simulink model "battery_phfb_inv_single_phase"  (R2024b)
settings: Solver=ode1be  StartTime=0.0  StopTime=simlength  FixedStep=ts_sim  MaxStep=ts_sim
undefined symbols (not defined in the file): Adrso, Aresd, Bresd, Cresd, Crso, dead_time, DThs_init, fPWM_INV, fPWM_ZVS, frequency_grid, I_FS, Iout_dc_nom, ki_i_inv, ki_i_zvs, ki_pll, ki_v_inv, ki_v_zvs, kp_i_inv, kp_i_zvs, kp_pll, kp_v_inv, kp_v_zvs, Ldrso, LFu_dc, magnitude, n1, number_of_cells, Q, q1kalman, q1Kalman, q2kalman, q2Kalman, q3Kalman, RCFu_dc, Rkalman, rKalman, RLFu_dc, Rload, Tambient, tc, ts_inv, ts_zvs, tsample, v1_trafo, v2_trafo, V_FS, Vout_dc_nom, w, weigth
libraries: fl_lib x207, nesl_utility x105, ee_lib x26, cstblocks x7, single_phase_transformer_lib x4, lithium_ion_cell_lib x1, simulink x1
(part 1 of 8)
settings Model: SimulationMode=accelerator  Creator=LTNBDA  LastModifiedBy=dbagn
settings SolverCC: ZeroCrossControl=EnableAll  ZeroCrossAlgorithm=Adaptive  AlgebraicLoopSolver=TrustRegion  SolverResetMethod=Robust  AutoInsertRateTranBlk=on
settings DataIOCC: LimitDataPoints=on  MaxDataPoints=1  SaveFormat=Array  SignalLoggingSaveFormat=ModelDataLogs  SaveOutput=off  SignalLogging=off  DSMLogging=off  SaveTime=off  ReturnWorkspaceOutputs=off
settings OptimizationCC: ExpressionDepthLimit=2147483647  InitFltsAndDblsToZero=on  EfficientMapNaN2IntZero=off  LifeSpan=inf
settings DebuggingCC: SaveWithParameterizedLinksMsg=none  UnderspecifiedInitializationDetection=Classic  MergeDetectMultiDrivingBlocksExec=none  SignalResolutionControl=TryResolveAllWithWarning  SolverPrmCheckMsg=warning  MultiTaskDSMMsg=warning  MultiTaskCondExecSysMsg=none  MultiTaskRateTransMsg=warning  FcnCallInpInsideContextMsg=warning  StateNameClashWarn=warning  SFUnexpectedBacktrackingDiag=warning  SFNoUnconditionalDefaultTransitionDiag=warning  ArithmeticOperatorsInVariantConditions=warning
settings HardwareCC: ProdBitPerLong=64  ProdLargestAtomicFloat=None  ProdIntDivRoundTo=Undefined  ProdEndianess=Unspecified  ProdHWDeviceType=Generic->64-bit Embedded Processor (LP64)  TargetBitPerPointer=64  TargetBitPerSizeT=64  TargetBitPerPtrDiffT=64  TargetLongLongMode=on  TargetIntDivRoundTo=Zero  TargetEndianess=LittleEndian  TargetWordSize=64  TargetHWDeviceType=MATLAB Host  ProdEqTarget=off
settings ModelReferenceCC: EnableRefExpFcnMdlSchedulingChecks=on  PropagateSignalLabelsOutOfModel=off
settings SFSimCC: SimUseLocalCustomCode=off  CustomCodeUndefinedFunction=UseInterfaceOnly
settings RTWCC: RTWUseLocalCustomCode=off  GPUComputeCapability=3.5
settings CodeAppCC: MaxIdLength=128  StateflowObjectComments=on
settings GRTTargetCC: TargetLangStandard=C89/C90 (ANSI)  CombineOutputUpdateFcns=off  GRTInterface=on
settings ConfigComp: CovMetricSettings=dw  CovSaveCumulativeToWorkspaceVar=on  CovSaveSingleToWorkspaceVar=on  CovExternalEMLEnable=off
settings SimscapeCC: SimscapeNormalizeSystem=off

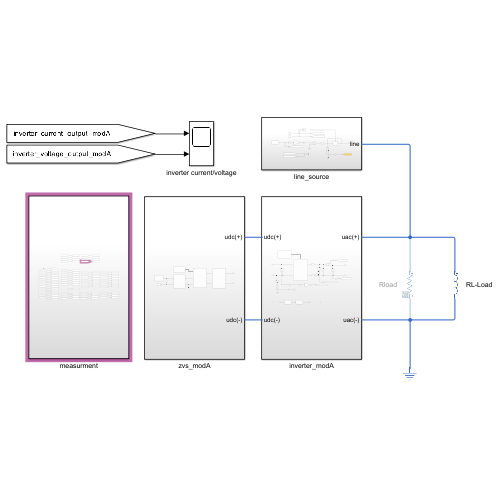
[thumbnail: Simulink's stored preview of the top-level diagram]
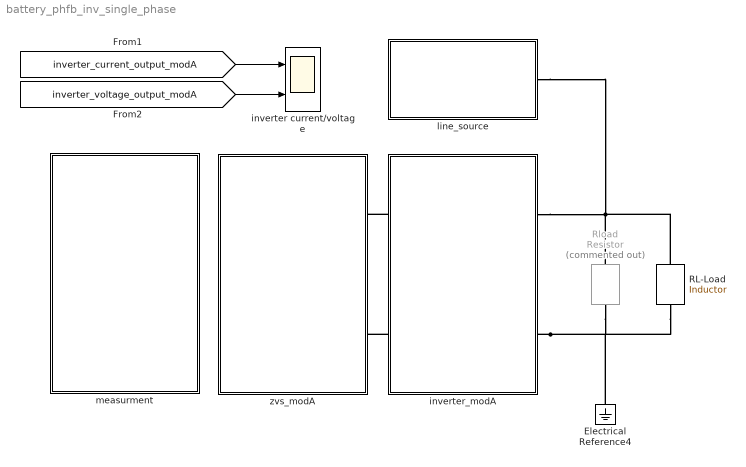
== system battery_phfb_inv_single_phase ==
  Electrical Reference4 : fl_lib/Electrical/Electrical Elements/Electrical Reference
  RL-Load : fl_lib/Electrical/Electrical Elements/Inductor  l=Lload H  r=Rload Ohm  g=1e-9 1/Ohm  i_specify=off  i_priority=None  i=0 A  i_nominal_specify=off  i_nominal_value=1  i_nominal_unit=A  v_specify=off  v_priority=None  v=0 V  v_nominal_specify=off  v_nominal_value=1  v_nominal_unit=V  i_L_specify=off  i_L_priority=High  i_L=0 A  i_L_nominal_specify=off  i_L_nominal_value=1  i_L_nominal_unit=A
  Rload : fl_lib/Electrical/Electrical Elements/Resistor  Commented=on  R=Rload Ohm  i_specify=off  i_priority=None  i=0 A  i_nominal_specify=off  i_nominal_value=1  i_nominal_unit=A  v_specify=off  v_priority=None  v=0 V  v_nominal_specify=off  v_nominal_value=1  v_nominal_unit=V
  inverter current/voltage : Scope  NumInputPorts=2
  inverter_modA : Subsystem
  line_source : Subsystem
  measurment : Subsystem
  zvs_modA : Subsystem
  wires:
  [inverter_current_output_modA] -> inverter current/voltage/1
  [inverter_voltage_output_modA] -> inverter current/voltage/2
  connections:
  inverter_modA/LConn2 -- zvs_modA/RConn2
  inverter_modA/LConn1 -- zvs_modA/RConn1
  inverter_modA/RConn1 -- RL-Load/LConn1 -- Rload/LConn1 -- line_source/LConn1
  inverter_modA/RConn2 -- RL-Load/RConn1 -- Rload/RConn1 -- Electrical Reference4/LConn1

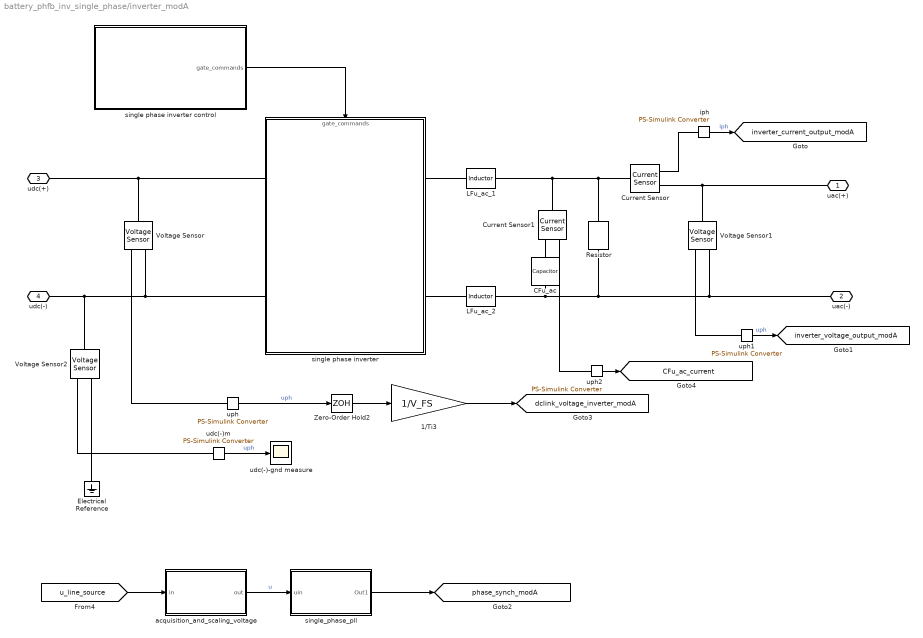
== system battery_phfb_inv_single_phase/inverter_modA ==
  1/Ti3 : Gain  Gain=1/V_FS  SaturateOnIntegerOverflow=on  OutDataTypeStr=Inherit: Same as input  ParamDataTypeStr=Inherit: Same as input
  CFu_ac : fl_lib/Electrical/Electrical Elements/Capacitor  c=CFu_ac F  r=RCFu_ac Ohm  g=0 1/Ohm  i_specify=off  i_priority=None  i=0 A  i_nominal_specify=off  i_nominal_value=1  i_nominal_unit=A  v_specify=off  v_priority=None  v=0 V  v_nominal_specify=off  v_nominal_value=1  v_nominal_unit=V  vc_specify=off  vc_priority=High  vc=0 V  vc_nominal_specify=off  vc_nominal_value=1  vc_nominal_unit=V
  Current Sensor : fl_lib/Electrical/Electrical Sensors/Current Sensor
  Current Sensor1 : fl_lib/Electrical/Electrical Sensors/Current Sensor
  Electrical Reference : fl_lib/Electrical/Electrical Elements/Electrical Reference
  LFu_ac_1 : fl_lib/Electrical/Electrical Elements/Inductor  l=LFu_ac H  r=RLFu_ac Ohm  g=0 1/Ohm  i_specify=off  i_priority=None  i=0 A  i_nominal_specify=off  i_nominal_value=1  i_nominal_unit=A  v_specify=off  v_priority=None  v=0 V  v_nominal_specify=off  v_nominal_value=1  v_nominal_unit=V  i_L_specify=off  i_L_priority=High  i_L=0 A  i_L_nominal_specify=off  i_L_nominal_value=1  i_L_nominal_unit=A
  LFu_ac_2 : fl_lib/Electrical/Electrical Elements/Inductor  l=LFu_ac H  r=RLFu_ac Ohm  g=0 1/Ohm  i_specify=off  i_priority=None  i=0 A  i_nominal_specify=off  i_nominal_value=1  i_nominal_unit=A  v_specify=off  v_priority=None  v=0 V  v_nominal_specify=off  v_nominal_value=1  v_nominal_unit=V  i_L_specify=off  i_L_priority=High  i_L=0 A  i_L_nominal_specify=off  i_L_nominal_value=1  i_L_nominal_unit=A
  Resistor : fl_lib/Electrical/Electrical Elements/Resistor  R=10e3 Ohm  i_specify=off  i_priority=None  i=0 A  i_nominal_specify=off  i_nominal_value=1  i_nominal_unit=A  v_specify=off  v_priority=None  v=0 V  v_nominal_specify=off  v_nominal_value=1  v_nominal_unit=V
  Voltage Sensor : fl_lib/Electrical/Electrical Sensors/Voltage Sensor
  Voltage Sensor1 : fl_lib/Electrical/Electrical Sensors/Voltage Sensor
  Voltage Sensor2 : fl_lib/Electrical/Electrical Sensors/Voltage Sensor
  Zero-Order Hold2 : ZeroOrderHold  SampleTime=ts_zvs
  acquisition_and_scaling_voltage : Subsystem
  iph : nesl_utility/PS-Simulink Converter  PhysicalDomain=network_engine_domain  SubClassName=ps_output  LeftPortType=input  RightPortType=output  PseudoPeriodic=off  Frequencies=[]  VectorFormat=1-D array  Unit=A  AffineConversion=off
  single phase inverter : Subsystem
      settings: PortSchema="{\"entries\":[{\"content\":{\"sides\":[{\"content\":{\"connectorIds\":[\"LConn1\",\"LConn2\"]},\"type\":\"ConnectorPlacement.EquallySpacedRectSide\",\"uuid\":\"4fcf4fea-d38f-431b-8a91-be3ce9782faf\"},{\"content\":{\"connectorIds\":[\"RConn1\",\"RConn2\"],\"side\":\"RIGHT\"},\"type\":\"ConnectorPlacement.EquallySpacedRectSide\",\"uuid\":\"0aa56277-92e9-4e3b-84c7-43398254a4d8\"},{\"content\":{\"connectorIds\":[\"In1\"],\"side\":\"TOP\"},\"type\":\"ConnectorPlacement.EquallySpacedRectSide\",\"uuid\":\"5cd150dc-bcaf-4cd7-b2a8-3db203726730\"}]},\"type\":\"ConnectorPlacement.EquallySpacedConnector\",\"uuid\":\"bf8194c4-c327-4d40-bea4-f1e7617f80b4\"}],\"packageUris\":[\"http://schema.mathworks.com/mf0/Connector/R2020b\"],\"version\":\"1.0\"}"
  single phase inverter control : Subsystem
  single_phase_pll : Subsystem
  udc(-)-gnd measure : Scope
  udc(-)m : nesl_utility/PS-Simulink Converter  PhysicalDomain=network_engine_domain  SubClassName=ps_output  LeftPortType=input  RightPortType=output  PseudoPeriodic=off  Frequencies=[]  VectorFormat=1-D array  Unit=V  AffineConversion=off
  uph : nesl_utility/PS-Simulink Converter  PhysicalDomain=network_engine_domain  SubClassName=ps_output  LeftPortType=input  RightPortType=output  PseudoPeriodic=off  Frequencies=[]  VectorFormat=1-D array  Unit=V  AffineConversion=off
  uph1 : nesl_utility/PS-Simulink Converter  PhysicalDomain=network_engine_domain  SubClassName=ps_output  LeftPortType=input  RightPortType=output  PseudoPeriodic=off  Frequencies=[]  VectorFormat=1-D array  Unit=V  AffineConversion=off
  uph2 : nesl_utility/PS-Simulink Converter  PhysicalDomain=network_engine_domain  SubClassName=ps_output  LeftPortType=input  RightPortType=output  PseudoPeriodic=off  Frequencies=[]  VectorFormat=1-D array  Unit=A  AffineConversion=off
  uac(+) : PMIOPort  Side=Right
  uac(-) : PMIOPort  Port=2  Side=Right
  udc(+) : PMIOPort  Port=3  Side=Left
  udc(-) : PMIOPort  Port=4  Side=Left
  tag scope: CFu_ac_current=global, dclink_voltage_inverter_modA=global, inverter_current_output_modA=global, inverter_voltage_output_modA=global, phase_synch_modA=global
  wires:
  single phase inverter control/1(gate_commands) -> single phase inverter/1(gate_commands)
  iph/1 -> [inverter_current_output_modA]  "iph"
  uph1/1 -> [inverter_voltage_output_modA]  "uph"
  uph2/1 -> [CFu_ac_current]
  acquisition_and_scaling_voltage/1(out) -> single_phase_pll/1(uin)  "u"
  single_phase_pll/1(Out1) -> [phase_synch_modA]
  [u_line_source] -> acquisition_and_scaling_voltage/1(in)
  uph/1 -> Zero-Order Hold2/1  "uph"
  Zero-Order Hold2/1 -> 1/Ti3/1
  udc(-)m/1 -> udc(-)-gnd measure/1  "uph"
  1/Ti3/1 -> [dclink_voltage_inverter_modA]
  connections:
  single phase inverter/RConn2 -- Voltage Sensor2/LConn1 -- udc(-)/RConn1 -- Voltage Sensor/RConn2
  single phase inverter/RConn1 -- Voltage Sensor/LConn1 -- udc(+)/RConn1
  LFu_ac_1/LConn1 -- single phase inverter/LConn1
  single phase inverter/LConn2 -- LFu_ac_2/RConn1
  Voltage Sensor1/RConn1 -- uph1/LConn1
  Resistor/LConn1 -- Current Sensor/LConn1 -- Current Sensor1/LConn1 -- LFu_ac_1/RConn1
  iph/LConn1 -- Current Sensor/RConn1
  Current Sensor/RConn2 -- uac(+)/RConn1 -- Voltage Sensor1/LConn1
  LFu_ac_2/LConn1 -- CFu_ac/RConn1 -- uac(-)/RConn1 -- Voltage Sensor1/RConn2 -- Resistor/RConn1
  Current Sensor1/RConn2 -- CFu_ac/LConn1
  Current Sensor1/RConn1 -- uph2/LConn1
  Electrical Reference/LConn1 -- Voltage Sensor2/RConn2
  Voltage Sensor2/RConn1 -- udc(-)m/LConn1
  Voltage Sensor/RConn1 -- uph/LConn1

== system battery_phfb_inv_single_phase/line_source ==
  Controlled Voltage Source : fl_lib/Electrical/Electrical Sources/Controlled Voltage Source
  Cos : Trigonometry  Operator=cos
  Electrical Reference : fl_lib/Electrical/Electrical Elements/Electrical Reference
  Electrical Reference1 : fl_lib/Electrical/Electrical Elements/Electrical Reference
  Gain : Gain  Gain=230*sqrt(2)
  Ld_grid : fl_lib/Electrical/Electrical Elements/Inductor  l=250e-6 H  r=3e-3 Ohm  g=0 1/Ohm  i_specify=off  i_priority=None  i=0 A  i_nominal_specify=off  i_nominal_value=1  i_nominal_unit=A  v_specify=off  v_priority=None  v=0 V  v_nominal_specify=off  v_nominal_value=1  v_nominal_unit=V  i_L_specify=off  i_L_priority=High  i_L=0 A  i_L_nominal_specify=off  i_L_nominal_value=1  i_L_nominal_unit=A
  Simulink-PS Converter : nesl_utility/Simulink-PS Converter  PhysicalDomain=network_engine_domain  SubClassName=ps_input  LeftPortType=input  RightPortType=output  PseudoPeriodic=off  Frequencies=[]  NoiseDistribution=none  NoiseParameters=[]  Unit=1  AffineConversion=off  FilteringAndDerivatives=provide  SimscapeFilterOrder=1  InputFilterTimeConstant=0.001  UdotUserProvided=0
  Step : Step  Time=2e3  After=15  SampleTime=0
  Step1 : Step  Time=1.2  Before=15  After=0  SampleTime=0
  Voltage Sensor2 : fl_lib/Electrical/Electrical Sensors/Voltage Sensor
  cmd_bypass_line/ups : Scope  NumInputPorts=2
  ideas_switch_based_switch1 : Subsystem
      settings: PortSchema="{\"entries\":[{\"content\":{\"sides\":[{\"content\":{\"connectorIds\":[\"LConn1\"]},\"type\":\"ConnectorPlacement.EquallySpacedRectSide\",\"uuid\":\"0c1d3d49-2b2f-458b-aa4f-29a8fc7e06a8\"},{\"content\":{\"connectorIds\":[\"RConn1\"],\"side\":\"RIGHT\"},\"type\":\"ConnectorPlacement.EquallySpacedRectSide\",\"uuid\":\"ca3eb42d-18fc-4989-b764-44975cb49bad\"},{\"content\":{\"connectorIds\":[\"In1\"],\"side\":\"TOP\"},\"type\":\"ConnectorPlacement.EquallySpacedRectSide\",\"uuid\":\"521c1188-cf36-48df-a46f-4a5e2a9fee19\"}]},\"type\":\"ConnectorPlacement.EquallySpacedConnector\",\"uuid\":\"019ba21c-6ae7-40bf-b23d-41e1cbba37d5\"}],\"packageUris\":[\"http://schema.mathworks.com/mf0/Connector/R2020b\"],\"version\":\"1.0\"}"
  phase_gen : Subsystem
  phase_grid/pll : Scope  NumInputPorts=2
  u_line_source : nesl_utility/PS-Simulink Converter  PhysicalDomain=network_engine_domain  SubClassName=ps_output  LeftPortType=input  RightPortType=output  PseudoPeriodic=off  Frequencies=[]  VectorFormat=1-D array  Unit=V  AffineConversion=off
  line : PMIOPort  Side=Left
  tag scope: cmd_bypass_line=global, cmd_bypass_ups=global, phase_grid=global, u_line_source=global
  wires:
  phase_gen/1(phase_gen) -> Cos/1, [phase_grid]
  Step1/1 -> cmd_bypass_line/ups/2, [cmd_bypass_ups]  "cmd_bypass_ups"
  Step/1 -> cmd_bypass_line/ups/1, [cmd_bypass_line]  "cmd_bypass_line"
  Cos/1 -> Gain/1
  Gain/1 -> Simulink-PS Converter/1
  [phase_synch_modA] -> phase_grid/pll/1  "phase_synch_modA"
  [phase_grid] -> phase_grid/pll/2  "phase_grid"
  [cmd_bypass_line] -> ideas_switch_based_switch1/1(gate_firing)
  u_line_source/1 -> [u_line_source]  "u_line_source"
  connections:
  Simulink-PS Converter/RConn1 -- Controlled Voltage Source/RConn1
  Electrical Reference/LConn1 -- Controlled Voltage Source/RConn2
  Controlled Voltage Source/LConn1 -- Ld_grid/LConn1
  Ld_grid/RConn1 -- ideas_switch_based_switch1/LConn1
  ideas_switch_based_switch1/RConn1 -- line/RConn1 -- Voltage Sensor2/LConn1
  Voltage Sensor2/RConn1 -- u_line_source/LConn1
  Electrical Reference1/LConn1 -- Voltage Sensor2/RConn2

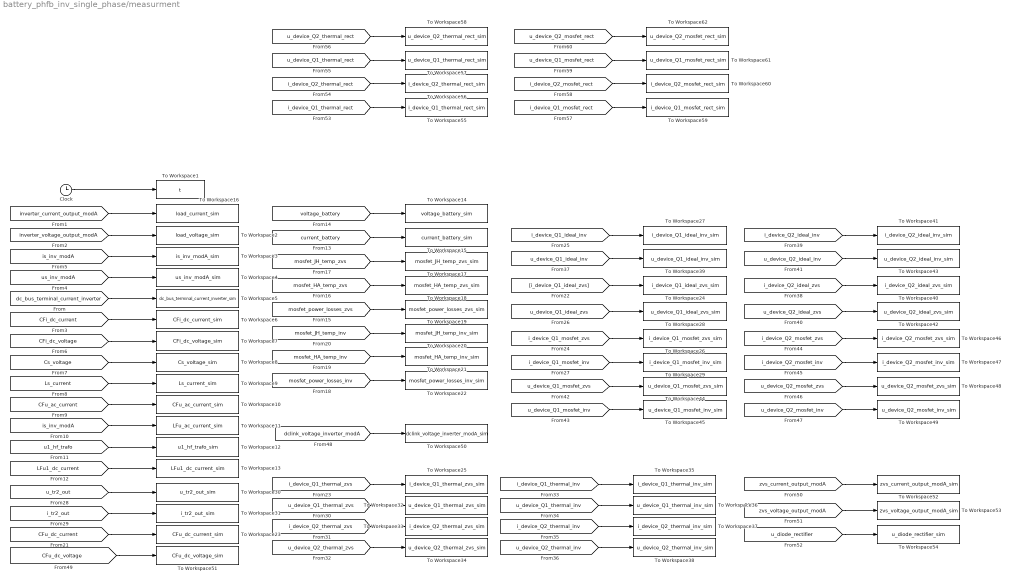
== system battery_phfb_inv_single_phase/measurment ==
  Clock : Clock
  To Workspace1 : ToWorkspace  VariableName=t  SampleTime=tc
      settings: MaxDataPoints=Nc
  To Workspace10 : ToWorkspace  VariableName=CFu_ac_current_sim  SampleTime=tc
      settings: MaxDataPoints=Nc
  To Workspace11 : ToWorkspace  VariableName=LFu_ac_current_sim  SampleTime=tc
      settings: MaxDataPoints=Nc
  To Workspace12 : ToWorkspace  VariableName=u1_hf_trafo_sim  SampleTime=tc
      settings: MaxDataPoints=Nc
  To Workspace13 : ToWorkspace  VariableName=LFu1_dc_current_sim  SampleTime=tc
      settings: MaxDataPoints=Nc
  To Workspace14 : ToWorkspace  VariableName=voltage_battery_sim  SampleTime=tc
      settings: MaxDataPoints=Nc
  To Workspace15 : ToWorkspace  VariableName=current_battery_sim  SampleTime=tc
      settings: MaxDataPoints=Nc
  To Workspace16 : ToWorkspace  VariableName=load_current_sim  SampleTime=tc
      settings: MaxDataPoints=Nc
  To Workspace17 : ToWorkspace  VariableName=mosfet_JH_temp_zvs_sim  SampleTime=tc
      settings: MaxDataPoints=Nc
  To Workspace18 : ToWorkspace  VariableName=mosfet_HA_temp_zvs_sim  SampleTime=tc
      settings: MaxDataPoints=Nc
  To Workspace19 : ToWorkspace  VariableName=mosfet_power_losses_zvs_sim  SampleTime=tc
      settings: MaxDataPoints=Nc
  To Workspace2 : ToWorkspace  VariableName=load_voltage_sim  SampleTime=tc
      settings: MaxDataPoints=Nc
  To Workspace20 : ToWorkspace  VariableName=mosfet_JH_temp_inv_sim  SampleTime=tc
      settings: MaxDataPoints=Nc
  To Workspace21 : ToWorkspace  VariableName=mosfet_HA_temp_inv_sim  SampleTime=tc
      settings: MaxDataPoints=Nc
  To Workspace22 : ToWorkspace  VariableName=mosfet_power_losses_inv_sim  SampleTime=tc
      settings: MaxDataPoints=Nc
  To Workspace23 : ToWorkspace  VariableName=CFu_dc_current_sim  SampleTime=tc
      settings: MaxDataPoints=Nc
  To Workspace24 : ToWorkspace  VariableName=i_device_Q1_ideal_zvs_sim  SampleTime=tc
      settings: MaxDataPoints=Nc
  To Workspace25 : ToWorkspace  VariableName=i_device_Q1_thermal_zvs_sim  SampleTime=tc
      settings: MaxDataPoints=Nc
  To Workspace26 : ToWorkspace  VariableName=i_device_Q1_mosfet_zvs_sim  SampleTime=tc
      settings: MaxDataPoints=Nc
  To Workspace27 : ToWorkspace  VariableName=i_device_Q1_ideal_inv_sim  SampleTime=tc
      settings: MaxDataPoints=Nc
  To Workspace28 : ToWorkspace  VariableName=u_device_Q1_ideal_zvs_sim  SampleTime=tc
      settings: MaxDataPoints=Nc
  To Workspace29 : ToWorkspace  VariableName=i_device_Q1_mosfet_inv_sim  SampleTime=tc
      settings: MaxDataPoints=Nc
  To Workspace3 : ToWorkspace  VariableName=is_inv_modA_sim  SampleTime=tc
      settings: MaxDataPoints=Nc
  To Workspace30 : ToWorkspace  VariableName=u_tr2_out_sim  SampleTime=tc
      settings: MaxDataPoints=Nc
  To Workspace31 : ToWorkspace  VariableName=i_tr2_out_sim  SampleTime=tc
      settings: MaxDataPoints=Nc
  To Workspace32 : ToWorkspace  VariableName=u_device_Q1_thermal_zvs_sim  SampleTime=tc
      settings: MaxDataPoints=Nc
  To Workspace33 : ToWorkspace  VariableName=i_device_Q2_thermal_zvs_sim  SampleTime=tc
      settings: MaxDataPoints=Nc
  To Workspace34 : ToWorkspace  VariableName=u_device_Q2_thermal_zvs_sim  SampleTime=tc
      settings: MaxDataPoints=Nc
  To Workspace35 : ToWorkspace  VariableName=i_device_Q1_thermal_inv_sim  SampleTime=tc
      settings: MaxDataPoints=Nc
  To Workspace36 : ToWorkspace  VariableName=u_device_Q1_thermal_inv_sim  SampleTime=tc
      settings: MaxDataPoints=Nc
  To Workspace37 : ToWorkspace  VariableName=i_device_Q2_thermal_inv_sim  SampleTime=tc
      settings: MaxDataPoints=Nc
  To Workspace38 : ToWorkspace  VariableName=u_device_Q2_thermal_inv_sim  SampleTime=tc
      settings: MaxDataPoints=Nc
  To Workspace39 : ToWorkspace  VariableName=u_device_Q1_ideal_inv_sim  SampleTime=tc
      settings: MaxDataPoints=Nc
  To Workspace4 : ToWorkspace  VariableName=us_inv_modA_sim  SampleTime=tc
      settings: MaxDataPoints=Nc
  To Workspace40 : ToWorkspace  VariableName=i_device_Q2_ideal_zvs_sim  SampleTime=tc
      settings: MaxDataPoints=Nc
  To Workspace41 : ToWorkspace  VariableName=i_device_Q2_ideal_inv_sim  SampleTime=tc
      settings: MaxDataPoints=Nc
  To Workspace42 : ToWorkspace  VariableName=u_device_Q2_ideal_zvs_sim  SampleTime=tc
      settings: MaxDataPoints=Nc
  To Workspace43 : ToWorkspace  VariableName=u_device_Q2_ideal_inv_sim  SampleTime=tc
      settings: MaxDataPoints=Nc
  To Workspace44 : ToWorkspace  VariableName=u_device_Q1_mosfet_zvs_sim  SampleTime=tc
      settings: MaxDataPoints=Nc
  To Workspace45 : ToWorkspace  VariableName=u_device_Q1_mosfet_inv_sim  SampleTime=tc
      settings: MaxDataPoints=Nc
  To Workspace46 : ToWorkspace  VariableName=i_device_Q2_mosfet_zvs_sim  SampleTime=tc
      settings: MaxDataPoints=Nc
  To Workspace47 : ToWorkspace  VariableName=i_device_Q2_mosfet_inv_sim  SampleTime=tc
      settings: MaxDataPoints=Nc
  To Workspace48 : ToWorkspace  VariableName=u_device_Q2_mosfet_zvs_sim  SampleTime=tc
      settings: MaxDataPoints=Nc
  To Workspace49 : ToWorkspace  VariableName=u_device_Q2_mosfet_inv_sim  SampleTime=tc
      settings: MaxDataPoints=Nc
  To Workspace5 : ToWorkspace  VariableName=dc_bus_terminal_current_inverter_sim  SampleTime=tc
      settings: MaxDataPoints=Nc
  To Workspace50 : ToWorkspace  VariableName=dclink_voltage_inverter_modA_sim  SampleTime=tc
      settings: MaxDataPoints=Nc
  To Workspace51 : ToWorkspace  VariableName=CFu_dc_voltage_sim  SampleTime=tc
      settings: MaxDataPoints=Nc
  To Workspace52 : ToWorkspace  VariableName=zvs_current_output_modA_sim  SampleTime=tc
      settings: MaxDataPoints=Nc
  To Workspace53 : ToWorkspace  VariableName=zvs_voltage_output_modA_sim  SampleTime=tc
      settings: MaxDataPoints=Nc
  To Workspace54 : ToWorkspace  VariableName=u_diode_rectifier_sim  SampleTime=tc
      settings: MaxDataPoints=Nc
  To Workspace55 : ToWorkspace  VariableName=i_device_Q1_thermal_rect_sim  SampleTime=tc
      settings: MaxDataPoints=Nc
  To Workspace56 : ToWorkspace  VariableName=i_device_Q2_thermal_rect_sim  SampleTime=tc
      settings: MaxDataPoints=Nc
  To Workspace57 : ToWorkspace  VariableName=u_device_Q1_thermal_rect_sim  SampleTime=tc
      settings: MaxDataPoints=Nc
  To Workspace58 : ToWorkspace  VariableName=u_device_Q2_thermal_rect_sim  SampleTime=tc
      settings: MaxDataPoints=Nc
  To Workspace59 : ToWorkspace  VariableName=i_device_Q1_mosfet_rect_sim  SampleTime=tc
      settings: MaxDataPoints=Nc
  To Workspace6 : ToWorkspace  VariableName=CFi_dc_current_sim  SampleTime=tc
      settings: MaxDataPoints=Nc
  To Workspace60 : ToWorkspace  VariableName=i_device_Q2_mosfet_rect_sim  SampleTime=tc
      settings: MaxDataPoints=Nc
  To Workspace61 : ToWorkspace  VariableName=u_device_Q1_mosfet_rect_sim  SampleTime=tc
      settings: MaxDataPoints=Nc
  To Workspace62 : ToWorkspace  VariableName=u_device_Q2_mosfet_rect_sim  SampleTime=tc
      settings: MaxDataPoints=Nc
  To Workspace7 : ToWorkspace  VariableName=CFi_dc_voltage_sim  SampleTime=tc
      settings: MaxDataPoints=Nc
  To Workspace8 : ToWorkspace  VariableName=Cs_voltage_sim  SampleTime=tc
      settings: MaxDataPoints=Nc
  To Workspace9 : ToWorkspace  VariableName=Ls_current_sim  SampleTime=tc
      settings: MaxDataPoints=Nc
  wires:
  Clock/1 -> To Workspace1/1
  [inverter_current_output_modA] -> To Workspace16/1
  [inverter_voltage_output_modA] -> To Workspace2/1
  [is_inv_modA] -> To Workspace3/1
  [us_inv_modA] -> To Workspace4/1
  [dc_bus_terminal_current_inverter] -> To Workspace5/1
  [CFi_dc_current] -> To Workspace6/1
  [CFi_dc_voltage] -> To Workspace7/1
  [Cs_voltage] -> To Workspace8/1
  [Ls_current] -> To Workspace9/1
  [CFu_ac_current] -> To Workspace10/1
  [is_inv_modA] -> To Workspace11/1
  [u1_hf_trafo] -> To Workspace12/1
  [LFu1_dc_current] -> To Workspace13/1
  [voltage_battery] -> To Workspace14/1
  [current_battery] -> To Workspace15/1
  [mosfet_JH_temp_zvs] -> To Workspace17/1
  [mosfet_HA_temp_zvs] -> To Workspace18/1
  [mosfet_power_losses_zvs] -> To Workspace19/1
  [mosfet_power_losses_inv] -> To Workspace22/1
  [mosfet_HA_temp_inv] -> To Workspace21/1
  [mosfet_JH_temp_inv] -> To Workspace20/1
  [CFu_dc_current] -> To Workspace23/1
  [i_device_Q1_ideal_zvs] -> To Workspace24/1
  [i_device_Q1_thermal_zvs] -> To Workspace25/1
  [i_device_Q1_mosfet_zvs] -> To Workspace26/1
  [i_device_Q1_mosfet_inv] -> To Workspace29/1
  [i_device_Q1_ideal_inv] -> To Workspace27/1
  [u_tr2_out] -> To Workspace30/1
  [i_tr2_out] -> To Workspace31/1
  [u_device_Q1_thermal_zvs] -> To Workspace32/1
  [u_device_Q2_thermal_zvs] -> To Workspace34/1
  [i_device_Q2_thermal_zvs] -> To Workspace33/1
  [i_device_Q2_thermal_inv] -> To Workspace37/1
  [u_device_Q2_thermal_inv] -> To Workspace38/1
  [u_device_Q1_thermal_inv] -> To Workspace36/1
  [i_device_Q1_thermal_inv] -> To Workspace35/1
  [u_device_Q1_ideal_zvs] -> To Workspace28/1
  [u_device_Q1_ideal_inv] -> To Workspace39/1
  [u_device_Q2_ideal_inv] -> To Workspace43/1
  [u_device_Q2_ideal_zvs] -> To Workspace42/1
  [i_device_Q2_ideal_inv] -> To Workspace41/1
  [i_device_Q2_ideal_zvs] -> To Workspace40/1
  [u_device_Q1_mosfet_inv] -> To Workspace45/1
  [u_device_Q1_mosfet_zvs] -> To Workspace44/1
  [u_device_Q2_mosfet_zvs] -> To Workspace48/1
  [u_device_Q2_mosfet_inv] -> To Workspace49/1
  [i_device_Q2_mosfet_inv] -> To Workspace47/1
  [i_device_Q2_mosfet_zvs] -> To Workspace46/1
  [dclink_voltage_inverter_modA] -> To Workspace50/1
  [CFu_dc_voltage] -> To Workspace51/1
  [zvs_voltage_output_modA] -> To Workspace53/1
  [zvs_current_output_modA] -> To Workspace52/1
  [u_diode_rectifier] -> To Workspace54/1
  [i_device_Q1_thermal_rect] -> To Workspace55/1
  [i_device_Q2_thermal_rect] -> To Workspace56/1
  [u_device_Q2_thermal_rect] -> To Workspace58/1
  [u_device_Q1_thermal_rect] -> To Workspace57/1
  [u_device_Q1_mosfet_rect] -> To Workspace61/1
  [u_device_Q2_mosfet_rect] -> To Workspace62/1
  [i_device_Q2_mosfet_rect] -> To Workspace60/1
  [i_device_Q1_mosfet_rect] -> To Workspace59/1

== system battery_phfb_inv_single_phase/zvs_modA ==
  Electrical Reference : fl_lib/Electrical/Electrical Elements/Electrical Reference
  Solver Configuration : nesl_utility/Solver Configuration  PhysicalDomain=network_engine_domain  SubClassName=solver  LeftPortType=input  RightPortType=generic  Tones=[]  Harmonics=[]  SimulateNoise=off  Profile=off  UseLocalSampling=off  EnableSwitchedLinearOptims=on  FrequencyDomain=off  UseCCode=off  RelTol=0.001  AbsTol=0.001  MinStep=1e-09  ToWorkspace=off  RevertToSquareIcSolve=off  NumHomotopyIterations=100  PhasorMode=off  PhasorModeNumHarmonics=1  ConsistencySolver=NEWTON_FTOL  IndexReductionMethod=DerivativeReplacement  DoDC=on  ResidualTolerance=1e-09  ConsistencyTolSource=GLOBAL  ConsistencyAbsTol=0.001  ConsistencyRelTol=0.001  ConsistencyTolFactor=0.001  UseLocalSolver=on  LocalSolverChoice=NE_BACKWARD_EULER_ADVANCER  ResolveIndetEquations=on  FunctionEvalNumThread=1  LocalSolverSampleTime=ts_sim  DoFixedCost=on  MaxNonlinIter=3  MaxModeIter=2  ComputeImpulses=off  ImpulseIterations=2  LinearAlgebra=auto  LinearAlgebraNumThread=0  EquationFormulation=NE_TIME_EF  DelaysMemoryBudget=1024  AutomaticFiltering=on  FilteringTimeConstant=0.001  PartitionStorageMethod=AS_NEEDED  PartitionMemoryBudget=1024  PartitionMethod=ROBUST  MultibodyUseLocalSolver=off  MultibodyLocalSolverChoice=ODE1  MultibodyLocalSolverSampleTime=0.001
  Voltage Source : ee_lib/Sources/Voltage Source  Commented=on  dc_voltage=90 V  ac_voltage=0 V  ac_shift=0 rad  ac_frequency=60 Hz  noise_mode=ee.enum.sources.noise.Disabled  PSD=0 V^2/Hz  sample_time=1e-3 s  repeatability=ee.enum.sources.repeatability.NotRepeatable  user_seed=0  auto_seed=3499211588  i_specify=off  i_priority=None  i=0 A  i_nominal_specify=off  i_nominal_value=1  i_nominal_unit=A  v_specify=off  v_priority=None  v=0 V  v_nominal_specify=off  v_nominal_value=1  v_nominal_unit=V
  battery_system : Subsystem
  dc/dc with galvanic isolation : Subsystem
  single_phase_ui_measure1 : Subsystem
  ui_measure : Subsystem
  zvs_ctrl : Subsystem
  udc(+) : PMIOPort  Side=Right
  udc(-) : PMIOPort  Port=2  Side=Right
  wires:
  zvs_ctrl/1(gate_commands) -> dc/dc with galvanic isolation/1(gate_commands)
  connections:
  dc/dc with galvanic isolation/RConn1 -- ui_measure/LConn1
  dc/dc with galvanic isolation/RConn2 -- ui_measure/LConn2
  udc(+)/RConn1 -- ui_measure/RConn1
  udc(-)/RConn1 -- ui_measure/RConn2
  dc/dc with galvanic isolation/LConn2 -- single_phase_ui_measure1/RConn2 -- Electrical Reference/LConn1
  battery_system/RConn1 -- Voltage Source/LConn1 -- single_phase_ui_measure1/LConn1
  single_phase_ui_measure1/RConn1 -- dc/dc with galvanic isolation/LConn1
  single_phase_ui_measure1/LConn2 -- Voltage Source/RConn1 -- Solver Configuration/RConn1

== system battery_phfb_inv_single_phase/inverter_modA/acquisition_and_scaling_voltage ==
  in : Inport
  1/Ti1 : Gain  Gain=1/V_FS  SaturateOnIntegerOverflow=on  OutDataTypeStr=Inherit: Same as input  ParamDataTypeStr=Inherit: Same as input
  Unit Delay4 : UnitDelay  SampleTime=ts_inv  HasFrameUpgradeWarning=on
  Zero-Order Hold2 : ZeroOrderHold  SampleTime=ts_inv
  out : Outport
  wires:
  1/Ti1/1 -> Unit Delay4/1
  Zero-Order Hold2/1 -> 1/Ti1/1
  Unit Delay4/1 -> out/1
  in/1 -> Zero-Order Hold2/1

== system battery_phfb_inv_single_phase/inverter_modA/single phase inverter ==
  gate_commands : Inport
  Current Sensor : fl_lib/Electrical/Electrical Sensors/Current Sensor
  HBridgeIdeal : Subsystem  Commented=on
  HBridgeMosfet : Subsystem
  HBridgeThermal : Subsystem  Commented=on
  Voltage Sensor1 : fl_lib/Electrical/Electrical Sensors/Voltage Sensor
  iph : nesl_utility/PS-Simulink Converter  PhysicalDomain=network_engine_domain  SubClassName=ps_output  LeftPortType=input  RightPortType=output  PseudoPeriodic=off  Frequencies=[]  VectorFormat=1-D array  Unit=A  AffineConversion=off
  uph1 : nesl_utility/PS-Simulink Converter  PhysicalDomain=network_engine_domain  SubClassName=ps_output  LeftPortType=input  RightPortType=output  PseudoPeriodic=off  Frequencies=[]  VectorFormat=1-D array  Unit=V  AffineConversion=off
  uac_out(+) : PMIOPort  Side=Left
  uac_out(-) : PMIOPort  Port=2  Side=Left
  udc(+) : PMIOPort  Port=3  Side=Right
  udc(-) : PMIOPort  Port=4  Side=Right
  tag scope: is_inv_modA=global, us_inv_modA=global
  wires:
  iph/1 -> [is_inv_modA]  "iph"
  uph1/1 -> [us_inv_modA]  "uph"
  gate_commands/1 -> HBridgeMosfet/1(gate_commands)
  connections:
  Current Sensor/RConn1 -- iph/LConn1
  Current Sensor/RConn2 -- Voltage Sensor1/LConn1 -- uac_out(+)/RConn1
  Voltage Sensor1/RConn1 -- uph1/LConn1
  Voltage Sensor1/RConn2 -- HBridgeMosfet/RConn2 -- uac_out(-)/RConn1
  HBridgeMosfet/LConn1 -- udc(+)/RConn1
  HBridgeMosfet/RConn1 -- Current Sensor/LConn1
  HBridgeMosfet/LConn2 -- udc(-)/RConn1

== system battery_phfb_inv_single_phase/inverter_modA/single phase inverter control ==
  Bus Creator : BusCreator  Inputs=4
  Bus Creator1 : BusCreator  Inputs=3
  Bus Creator2 : BusCreator  Inputs=2
  acquisition_and_scaling_current : Subsystem
  acquisition_and_scaling_voltage : Subsystem
  dqbased_single_phase_inverter_ctrl : Subsystem  Commented=on
  is/is_ref : Scope  NumInputPorts=3
  pwm : Subsystem
  references_generator : Subsystem
  rpi_based_single_phase_inverter_ctrl : Subsystem
  gate_commands : Outport
  wires:
  pwm/3(m2_top) -> Bus Creator/3
  Bus Creator/1 -> gate_commands/1
  pwm/1(m1_top) -> Bus Creator/1
  pwm/2(m1_bottom) -> Bus Creator/2
  pwm/4(m2_bottom) -> Bus Creator/4
  [is_inv_modA] -> acquisition_and_scaling_current/1(in)
  [inverter_voltage_output_modA] -> acquisition_and_scaling_voltage/1(in)
  acquisition_and_scaling_current/1(out) -> rpi_based_single_phase_inverter_ctrl/1(i_out_inverter_pu)  "is_pu"
  acquisition_and_scaling_voltage/1(out) -> rpi_based_single_phase_inverter_ctrl/2(u_out_inverter_pu)  "u_out_inverter_pu"
  rpi_based_single_phase_inverter_ctrl/1(u_ctrl_out) -> is/is_ref/3, pwm/1(vout)  "u_ctrl_out"
  references_generator/1(i_out_inverter_reference_pu) -> rpi_based_single_phase_inverter_ctrl/3(i_out_inverter_reference_pu)  "is_ref_pu"
  references_generator/2(u_out_inverter_reference_pu) -> rpi_based_single_phase_inverter_ctrl/4(u_out_inverter_reference_pu)  "u_out_inverter_reference_pu"
  Bus Creator1/1 -> is/is_ref/2  "is_tracking"
  [is_inv_modA] -> Bus Creator2/2  "is"
  Bus Creator2/1 -> is/is_ref/1  "load"
  [inverter_voltage_output_modA] -> Bus Creator2/1  "u_out"
  [i_out_inverter_pu_ref] -> Bus Creator1/2  "i_out_inverter_pu_ref"
  [i_out_inverter_pu] -> Bus Creator1/3  "i_out_inverter_pu"
  [id_inv_pu_ref] -> Bus Creator1/1  "id_inv_pu_ref"

== system battery_phfb_inv_single_phase/inverter_modA/single_phase_pll ==
  uin : Inport
  Constant : Constant  Value=2*pi*frequency_grid
  Constant2 : Constant  Value=0
  Sum : Sum  Inputs=|++
  Sum1 : Sum  Inputs=|++
  Terminator1 : Terminator
  Terminator2 : Terminator
  Terminator3 : Terminator
  Unit Delay1 : UnitDelay  SampleTime=ts_inv  HasFrameUpgradeWarning=on
  alphabeta2xieta : MATLAB Function  TreatAsAtomicUnit=on  SystemSampleTime=ts_inv
  double_integrator_observer : Subsystem
  freq_pll : Gain  Gain=1/2/pi
  omega_int_ts : Gain  Gain=ts_inv
  pi-ctrl : Subsystem  mask{kp=kp_pll, ki=ki_pll, ts=ts_inv, sat_pos=2*pi*frequency_grid, sat_neg=-2*pi*frequency_grid}
  theta_pll_hat : Gain
  ualpha_pll : Gain
  ubeta_pll : Gain
  ueta_pll : Gain  Gain=-1
  ueta_pll_flt : cstblocks/LTI System  sys=Hd  IC=[]  PadeOrder=0
  uxi_pll : Gain
  uxi_pll_flt : cstblocks/LTI System  sys=Hd  IC=[]  PadeOrder=0
  xieta2alphabeta : MATLAB Function  TreatAsAtomicUnit=on  SystemSampleTime=ts_inv
  Out1 : Outport
  wires:
  Sum/1 -> double_integrator_observer/1(theta), xieta2alphabeta/3(gamma), alphabeta2xieta/3(gamma), Unit Delay1/1
  Unit Delay1/1 -> Sum/2
  alphabeta2xieta/1(xi) -> uxi_pll_flt/1, uxi_pll/1
  xieta2alphabeta/2(beta) -> ubeta_pll/1
  alphabeta2xieta/2(eta) -> ueta_pll_flt/1, ueta_pll/1
  omega_int_ts/1 -> Sum/1
  double_integrator_observer/1(theta_hat) -> theta_pll_hat/1  "theta_hat"
  uin/1 -> alphabeta2xieta/1(alpha)
  freq_pll/1 -> Terminator1/1  "freq_pll"
  ueta_pll_flt/1 -> xieta2alphabeta/2(eta)
  uxi_pll_flt/1 -> xieta2alphabeta/1(xi)
  ueta_pll/1 -> pi-ctrl/1(x)
  Sum1/1 -> freq_pll/1, omega_int_ts/1  "freq_pll"
  Constant2/1 -> pi-ctrl/2(xref)
  uxi_pll/1 -> Terminator2/1
  ubeta_pll/1 -> alphabeta2xieta/2(beta)
  xieta2alphabeta/1(alpha) -> ualpha_pll/1
  ualpha_pll/1 -> Terminator3/1
  pi-ctrl/1(u) -> Sum1/1
  Constant/1 -> Sum1/2
  theta_pll_hat/1 -> Out1/1  "theta_pll_hat"

== system battery_phfb_inv_single_phase/line_source/ideas_switch_based_switch1 ==
  gate_firing : Inport
  Simulink-PS Converter : nesl_utility/Simulink-PS Converter  PhysicalDomain=network_engine_domain  SubClassName=ps_input  LeftPortType=input  RightPortType=output  PseudoPeriodic=off  Frequencies=[]  NoiseDistribution=none  NoiseParameters=[]  Unit=1  AffineConversion=off  FilteringAndDerivatives=provide  SimscapeFilterOrder=1  InputFilterTimeConstant=0.001  UdotUserProvided=0
  Switch : fl_lib/Electrical/Electrical Elements/Switch  R_closed=Ron Ohm  G_open=1e-8 1/Ohm  Threshold=7.5  i_specify=off  i_priority=None  i=0 A  i_nominal_specify=off  i_nominal_value=1  i_nominal_unit=A  v_specify=off  v_priority=None  v=0 V  v_nominal_specify=off  v_nominal_value=1  v_nominal_unit=V
  u1 : PMIOPort  Side=Left
  u2 : PMIOPort  Port=2  Side=Right
  wires:
  gate_firing/1 -> Simulink-PS Converter/1
  connections:
  Simulink-PS Converter/RConn1 -- Switch/RConn1
  Switch/LConn1 -- u2/RConn1
  u1/RConn1 -- Switch/RConn2

== system battery_phfb_inv_single_phase/line_source/phase_gen ==
  Constant4 : Constant  Value=2*pi*frequency_grid
  Sum4 : Sum  SaturateOnIntegerOverflow=on
  Unit Delay1 : UnitDelay  SampleTime=ts_inv  HasFrameUpgradeWarning=on
  bounder1 : MATLAB Function  TreatAsAtomicUnit=on  SystemSampleTime=ts_inv
  kp2 : Gain  Gain=ts_inv  SaturateOnIntegerOverflow=on  OutDataTypeStr=Inherit: Same as input  ParamDataTypeStr=Inherit: Same as input
  phase_gen : Outport  VectorParamsAs1DForOutWhenUnconnected=off
  wires:
  bounder1/1(y) -> Unit Delay1/1  "grid_emu_phase"
  kp2/1 -> Sum4/1
  Constant4/1 -> kp2/1
  Unit Delay1/1 -> Sum4/2, phase_gen/1
  Sum4/1 -> bounder1/1(u)

== system battery_phfb_inv_single_phase/zvs_modA/battery_system ==
  Electrical Reference1 : fl_lib/Electrical/Electrical Elements/Electrical Reference
  LithiumIonBattery : Subsystem
  Uout+ : PMIOPort  Side=Right
  connections:
  LithiumIonBattery/RConn2 -- Electrical Reference1/LConn1
  LithiumIonBattery/RConn1 -- Uout+/RConn1

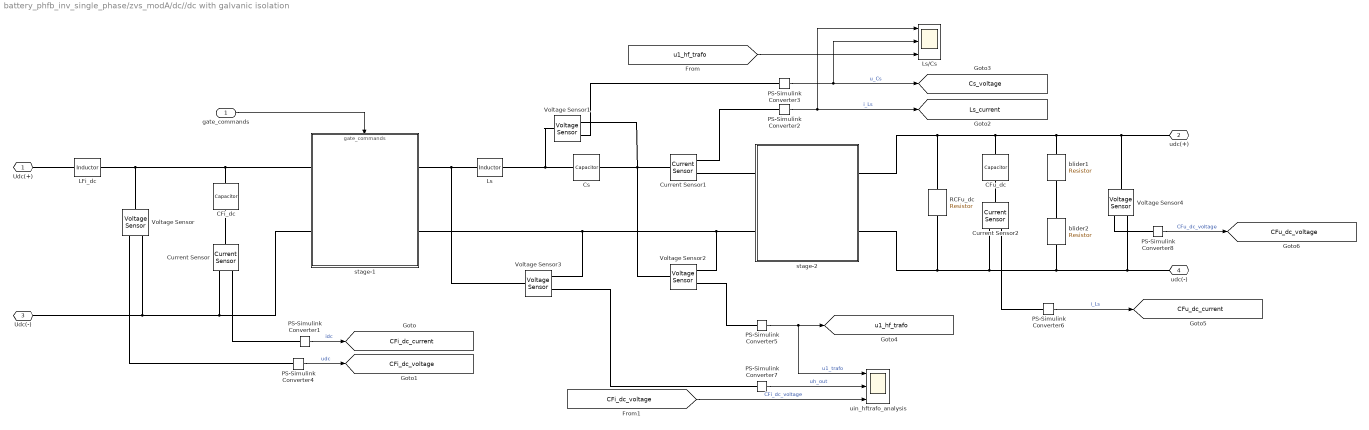
== system battery_phfb_inv_single_phase/zvs_modA/dc//dc with galvanic isolation ==
  gate_commands : Inport
  CFi_dc : fl_lib/Electrical/Electrical Elements/Capacitor  c=CFi_dc F  r=RCFi_dc_internal Ohm  g=0 1/Ohm  i_specify=off  i_priority=None  i=0 A  i_nominal_specify=off  i_nominal_value=1  i_nominal_unit=A  v_specify=off  v_priority=None  v=0 V  v_nominal_specify=off  v_nominal_value=1  v_nominal_unit=V  vc_specify=off  vc_priority=High  vc=0 V  vc_nominal_specify=off  vc_nominal_value=1  vc_nominal_unit=V
  CFu_dc : fl_lib/Electrical/Electrical Elements/Capacitor  c=CFu_dc F  r=RCFu_dc_internal Ohm  g=0 1/Ohm  i_specify=off  i_priority=None  i=0 A  i_nominal_specify=off  i_nominal_value=1  i_nominal_unit=A  v_specify=off  v_priority=None  v=0 V  v_nominal_specify=off  v_nominal_value=1  v_nominal_unit=V  vc_specify=off  vc_priority=High  vc=0 V  vc_nominal_specify=off  vc_nominal_value=1  vc_nominal_unit=V
  Cs : fl_lib/Electrical/Electrical Elements/Capacitor  c=Cs F  r=1e-6 Ohm  g=0 1/Ohm  i_specify=off  i_priority=None  i=0 A  i_nominal_specify=off  i_nominal_value=1  i_nominal_unit=A  v_specify=off  v_priority=None  v=0 V  v_nominal_specify=off  v_nominal_value=1  v_nominal_unit=V  vc_specify=off  vc_priority=High  vc=0 V  vc_nominal_specify=off  vc_nominal_value=1  vc_nominal_unit=V
  Current Sensor : fl_lib/Electrical/Electrical Sensors/Current Sensor
  Current Sensor1 : fl_lib/Electrical/Electrical Sensors/Current Sensor
  Current Sensor2 : fl_lib/Electrical/Electrical Sensors/Current Sensor
  LFi_dc : fl_lib/Electrical/Electrical Elements/Inductor  l=10e-6 H  r=0 Ohm  g=1e-9 1/Ohm  i_specify=off  i_priority=None  i=0 A  i_nominal_specify=off  i_nominal_value=1  i_nominal_unit=A  v_specify=off  v_priority=None  v=0 V  v_nominal_specify=off  v_nominal_value=1  v_nominal_unit=V  i_L_specify=off  i_L_priority=High  i_L=0 A  i_L_nominal_specify=off  i_L_nominal_value=1  i_L_nominal_unit=A
  Ls : fl_lib/Electrical/Electrical Elements/Inductor  l=Ls H  r=0 Ohm  g=1e-9 1/Ohm  i_specify=off  i_priority=None  i=0 A  i_nominal_specify=off  i_nominal_value=1  i_nominal_unit=A  v_specify=off  v_priority=None  v=0 V  v_nominal_specify=off  v_nominal_value=1  v_nominal_unit=V  i_L_specify=off  i_L_priority=High  i_L=0 A  i_L_nominal_specify=off  i_L_nominal_value=1  i_L_nominal_unit=A
  Ls/Cs : Scope  NumInputPorts=3
  PS-Simulink Converter1 : nesl_utility/PS-Simulink Converter  PhysicalDomain=network_engine_domain  SubClassName=ps_output  LeftPortType=input  RightPortType=output  PseudoPeriodic=off  Frequencies=[]  VectorFormat=1-D array  Unit=A  AffineConversion=on
  PS-Simulink Converter2 : nesl_utility/PS-Simulink Converter  PhysicalDomain=network_engine_domain  SubClassName=ps_output  LeftPortType=input  RightPortType=output  PseudoPeriodic=off  Frequencies=[]  VectorFormat=1-D array  Unit=A  AffineConversion=on
  PS-Simulink Converter{3..5,7..8} (5 alike) : nesl_utility/PS-Simulink Converter  PhysicalDomain=network_engine_domain  SubClassName=ps_output  LeftPortType=input  RightPortType=output  PseudoPeriodic=off  Frequencies=[]  VectorFormat=1-D array  Unit=V  AffineConversion=on
  PS-Simulink Converter6 : nesl_utility/PS-Simulink Converter  PhysicalDomain=network_engine_domain  SubClassName=ps_output  LeftPortType=input  RightPortType=output  PseudoPeriodic=off  Frequencies=[]  VectorFormat=1-D array  Unit=A  AffineConversion=on
  RCFu_dc : fl_lib/Electrical/Electrical Elements/Resistor  R=RCFu_dc Ohm  i_specify=off  i_priority=None  i=0 A  i_nominal_specify=off  i_nominal_value=1  i_nominal_unit=A  v_specify=off  v_priority=None  v=0 V  v_nominal_specify=off  v_nominal_value=1  v_nominal_unit=V
  Voltage Sensor{,1..4} (5 alike) : fl_lib/Electrical/Electrical Sensors/Voltage Sensor
  blider1 : fl_lib/Electrical/Electrical Elements/Resistor  R=1e4 Ohm  i_specify=off  i_priority=None  i=0 A  i_nominal_specify=off  i_nominal_value=1  i_nominal_unit=A  v_specify=off  v_priority=None  v=0 V  v_nominal_specify=off  v_nominal_value=1  v_nominal_unit=V
  blider2 : fl_lib/Electrical/Electrical Elements/Resistor  R=1e4 Ohm  i_specify=off  i_priority=None  i=0 A  i_nominal_specify=off  i_nominal_value=1  i_nominal_unit=A  v_specify=off  v_priority=None  v=0 V  v_nominal_specify=off  v_nominal_value=1  v_nominal_unit=V
  stage-1 : Subsystem
      settings: PortSchema="{\"entries\":[{\"content\":{\"sides\":[{\"content\":{\"connectorIds\":[\"LConn1\",\"LConn2\"]},\"type\":\"ConnectorPlacement.EquallySpacedRectSide\",\"uuid\":\"c872503a-61af-4937-bdf2-4de4f8645573\"},{\"content\":{\"connectorIds\":[\"RConn1\",\"RConn2\"],\"side\":\"RIGHT\"},\"type\":\"ConnectorPlacement.EquallySpacedRectSide\",\"uuid\":\"3b83f060-86a2-4569-84b5-d9f7c0485347\"},{\"content\":{\"connectorIds\":[\"In1\"],\"side\":\"TOP\"},\"type\":\"ConnectorPlacement.EquallySpacedRectSide\",\"uuid\":\"bf191d46-ce71-4d15-9dd0-24cc57253577\"}]},\"type\":\"ConnectorPlacement.EquallySpacedConnector\",\"uuid\":\"1b28ceee-25d0-45ae-a3c4-c2563f0d63ba\"}],\"packageUris\":[\"http://schema.mathworks.com/mf0/Connector/R2020b\"],\"version\":\"1.0\"}"
  stage-2 : Subsystem
  uin_hftrafo_analysis : Scope  NumInputPorts=3
  Udc(+) : PMIOPort  Side=Left
  udc(+) : PMIOPort  Port=2  Side=Right
  Udc(-) : PMIOPort  Port=3  Side=Left
  udc(-) : PMIOPort  Port=4  Side=Right
  tag scope: CFi_dc_current=global, CFi_dc_voltage=global, CFu_dc_current=global, CFu_dc_voltage=global, Cs_voltage=global, Ls_current=global, u1_hf_trafo=global
  wires:
  gate_commands/1 -> stage-1/1(gate_commands)
  PS-Simulink Converter1/1 -> [CFi_dc_current]  "idc"
  PS-Simulink Converter4/1 -> [CFi_dc_voltage]  "udc"
  PS-Simulink Converter2/1 -> Ls/Cs/1, [Ls_current]  "i_Ls"
  PS-Simulink Converter3/1 -> Ls/Cs/2, [Cs_voltage]  "u_Cs"
  PS-Simulink Converter5/1 -> uin_hftrafo_analysis/1, [u1_hf_trafo]  "u1_trafo"
  [u1_hf_trafo] -> Ls/Cs/3
  PS-Simulink Converter6/1 -> [CFu_dc_current]  "i_Ls"
  PS-Simulink Converter7/1 -> uin_hftrafo_analysis/2  "uh_out"
  [CFi_dc_voltage] -> uin_hftrafo_analysis/3  "CFi_dc_voltage"
  PS-Simulink Converter8/1 -> [CFu_dc_voltage]  "CFu_dc_voltage"
  connections:
  stage-2/LConn2 -- Voltage Sensor2/RConn2 -- Voltage Sensor3/RConn2 -- stage-1/LConn2
  stage-1/RConn1 -- CFi_dc/LConn1 -- Voltage Sensor/LConn1 -- LFi_dc/RConn1
  stage-1/RConn2 -- Current Sensor/RConn2 -- Voltage Sensor/RConn2 -- Udc(-)/RConn1
  stage-2/RConn2 -- Current Sensor2/RConn2 -- blider2/RConn1 -- udc(-)/RConn1 -- Voltage Sensor4/RConn2 -- RCFu_dc/RConn1
  blider2/LConn1 -- blider1/RConn1
  RCFu_dc/LConn1 -- stage-2/RConn1 -- udc(+)/RConn1 -- Voltage Sensor4/LConn1 -- blider1/LConn1 -- CFu_dc/LConn1
  LFi_dc/LConn1 -- Udc(+)/RConn1
  Current Sensor/LConn1 -- CFi_dc/RConn1
  Current Sensor/RConn1 -- PS-Simulink Converter1/LConn1
  PS-Simulink Converter4/LConn1 -- Voltage Sensor/RConn1
  stage-1/LConn1 -- Voltage Sensor3/LConn1 -- Ls/LConn1
  Current Sensor1/RConn2 -- stage-2/LConn1
  PS-Simulink Converter2/LConn1 -- Current Sensor1/RConn1
  Voltage Sensor1/RConn1 -- PS-Simulink Converter3/LConn1
  Voltage Sensor2/RConn1 -- PS-Simulink Converter5/LConn1
  Voltage Sensor1/RConn2 -- Cs/RConn1 -- Current Sensor1/LConn1 -- Voltage Sensor2/LConn1
  Ls/RConn1 -- Voltage Sensor1/LConn1 -- Cs/LConn1
  CFu_dc/RConn1 -- Current Sensor2/LConn1
  PS-Simulink Converter6/LConn1 -- Current Sensor2/RConn1
  Voltage Sensor3/RConn1 -- PS-Simulink Converter7/LConn1
  Voltage Sensor4/RConn1 -- PS-Simulink Converter8/LConn1

== system battery_phfb_inv_single_phase/zvs_modA/single_phase_ui_measure1 ==
  Bus Creator : BusCreator  Inputs=2
  Current Sensor : fl_lib/Electrical/Electrical Sensors/Current Sensor
  Selector : Selector  InputPortWidth=2  IndexOptions=Index vector (dialog)  Indices=2  OutputSizes=1
  Selector1 : Selector  InputPortWidth=2  IndexOptions=Index vector (dialog)  Indices=1  OutputSizes=1
  Voltage Sensor : fl_lib/Electrical/Electrical Sensors/Voltage Sensor
  input : Scope  NumInputPorts=2
  iph : nesl_utility/PS-Simulink Converter  PhysicalDomain=network_engine_domain  SubClassName=ps_output  LeftPortType=input  RightPortType=output  PseudoPeriodic=off  Frequencies=[]  VectorFormat=1-D array  Unit=A  AffineConversion=off
  uph : nesl_utility/PS-Simulink Converter  PhysicalDomain=network_engine_domain  SubClassName=ps_output  LeftPortType=input  RightPortType=output  PseudoPeriodic=off  Frequencies=[]  VectorFormat=1-D array  Unit=V  AffineConversion=off
  Udc(+) : PMIOPort  Side=Left
  udc(+) : PMIOPort  Port=2  Side=Right
  Udc(-) : PMIOPort  Port=3  Side=Left
  udc(-) : PMIOPort  Port=4  Side=Right
  tag scope: current_battery=global, voltage_battery=global
  wires:
  Bus Creator/1 -> Selector/1, Selector1/1  "ui_data"
  iph/1 -> Bus Creator/1  "iph"
  uph/1 -> Bus Creator/2  "uph"
  Selector1/1 -> [current_battery], input/1  "current_battery"
  Selector/1 -> input/2, [voltage_battery]  "voltage_battery"
  connections:
  iph/LConn1 -- Current Sensor/RConn1
  Voltage Sensor/LConn1 -- Current Sensor/LConn1 -- Udc(+)/RConn1
  Current Sensor/RConn2 -- udc(+)/RConn1
  Voltage Sensor/RConn1 -- uph/LConn1
  Voltage Sensor/RConn2 -- Udc(-)/RConn1 -- udc(-)/RConn1

== system battery_phfb_inv_single_phase/zvs_modA/ui_measure ==
  Bus Creator : BusCreator  Inputs=2
  Current Sensor : fl_lib/Electrical/Electrical Sensors/Current Sensor
  Selector : Selector  InputPortWidth=2  IndexOptions=Index vector (dialog)  Indices=2  OutputSizes=1
  Selector1 : Selector  InputPortWidth=2  IndexOptions=Index vector (dialog)  Indices=1  OutputSizes=1
  Voltage Sensor : fl_lib/Electrical/Electrical Sensors/Voltage Sensor
  idc/udc zvs modA : Scope  NumInputPorts=2
  iph : nesl_utility/PS-Simulink Converter  PhysicalDomain=network_engine_domain  SubClassName=ps_output  LeftPortType=input  RightPortType=output  PseudoPeriodic=off  Frequencies=[]  VectorFormat=1-D array  Unit=A  AffineConversion=off
  uph : nesl_utility/PS-Simulink Converter  PhysicalDomain=network_engine_domain  SubClassName=ps_output  LeftPortType=input  RightPortType=output  PseudoPeriodic=off  Frequencies=[]  VectorFormat=1-D array  Unit=V  AffineConversion=off
  Udc(+) : PMIOPort  Side=Left
  udc(+) : PMIOPort  Port=2  Side=Right
  Udc(-) : PMIOPort  Port=3  Side=Left
  udc(-) : PMIOPort  Port=4  Side=Right
  tag scope: zvs_current_output_modA=global, zvs_voltage_output_modA=global
  wires:
  [zvs_current_output_modA] -> idc/udc zvs modA/1  "zvs_current_output_modA"
  [zvs_voltage_output_modA] -> idc/udc zvs modA/2  "zvs_voltage_output_modA"
  Selector1/1 -> [zvs_current_output_modA]
  Selector/1 -> [zvs_voltage_output_modA]
  Bus Creator/1 -> Selector/1, Selector1/1  "ui_data"
  iph/1 -> Bus Creator/1  "iph"
  uph/1 -> Bus Creator/2  "uph"
  connections:
  iph/LConn1 -- Current Sensor/RConn1
  Voltage Sensor/LConn1 -- Current Sensor/LConn1 -- Udc(+)/RConn1
  Current Sensor/RConn2 -- udc(+)/RConn1
  Voltage Sensor/RConn1 -- uph/LConn1
  Voltage Sensor/RConn2 -- Udc(-)/RConn1 -- udc(-)/RConn1

== system battery_phfb_inv_single_phase/zvs_modA/zvs_ctrl ==
  Bus Creator : BusCreator  Inputs=4
  modulator1 : Subsystem
  references : Subsystem
  sampling_i_filter1 : Subsystem
  sampling_v_filter1 : Subsystem
  sampling_v_filter2 : Subsystem
  vi ctrl : Subsystem
  gate_commands : Outport
  wires:
  [zvs_voltage_output_modA] -> sampling_v_filter1/1(in)
  [zvs_current_output_modA] -> sampling_i_filter1/1(in)
  vi ctrl/1(phase_displacement) -> modulator1/1(phase_displacement)
  sampling_i_filter1/1(out_pu) -> vi ctrl/1(iout)
  sampling_v_filter1/1(out_pu) -> vi ctrl/2(vout)
  sampling_v_filter2/1(out_pu) -> vi ctrl/3(vout_ref)
  references/1(vout_ref) -> sampling_v_filter2/1(in)
  Bus Creator/1 -> gate_commands/1
  modulator1/1(gate_Q1) -> Bus Creator/1
  modulator1/2(gate_Q2) -> Bus Creator/2
  modulator1/3(gate_Q3) -> Bus Creator/3
  modulator1/4(gate_Q4) -> Bus Creator/4
